simulink model "schemes"  (R2019b)
settings: Solver=VariableStepAuto  StartTime=0.0  StopTime=10.0  RelTol=1e-3
undefined symbols (not defined in the file): Ki, Kp
settings Model: Creator=joaotiagoalmeida  LastModifiedBy=joaotiagoalmeida

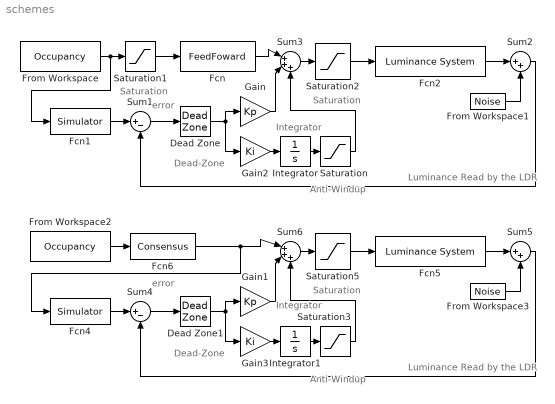
== system schemes ==
  note: Anti-Windup
  note: Dead-Zone
  note: Saturation
  note: Saturation
  note: error
  note: Luminance Read by the LDR
  note: Integrator
  note: error
  note: Luminance Read by the LDR
  note: Anti-Windup
  note: Saturation
  note: Dead-Zone
  note: Integrator
  Dead Zone : DeadZone  SaturateOnIntegerOverflow=on
  Dead Zone1 : DeadZone  SaturateOnIntegerOverflow=on
  Fcn : Fcn  Expr=FeedFoward
  Fcn1 : Fcn  Expr=Simulator
  Fcn2 : Fcn  Expr=Luminance System
  Fcn4 : Fcn  Expr=Simulator
  Fcn5 : Fcn  Expr=Luminance System
  Fcn6 : Fcn  Expr=Consensus
  From Workspace : FromWorkspace  VariableName=Occupancy  OutDataTypeStr=double  SampleTime=0  OutputAfterFinalValue=Cyclic repetition
  From Workspace1 : FromWorkspace  VariableName=Noise  OutDataTypeStr=double  SampleTime=0  OutputAfterFinalValue=Cyclic repetition
  From Workspace2 : FromWorkspace  VariableName=Occupancy  OutDataTypeStr=double  SampleTime=0  OutputAfterFinalValue=Cyclic repetition
  From Workspace3 : FromWorkspace  VariableName=Noise  OutDataTypeStr=double  SampleTime=0  OutputAfterFinalValue=Cyclic repetition
  Gain : Gain  Gain=Kp
  Gain1 : Gain  Gain=Kp
  Gain2 : Gain  Gain=Ki
  Gain3 : Gain  Gain=Ki
  Integrator : Integrator
  Integrator1 : Integrator
  Saturation{,1..3,5} (5 alike) : Saturate
  Sum1 : Sum  Inputs=|+-
  Sum2 : Sum  Inputs=|++
  Sum3 : Sum  Inputs=|+++
  Sum4 : Sum  Inputs=|+-
  Sum5 : Sum  Inputs=|++
  Sum6 : Sum  Inputs=|+++
  wires:
  Fcn1/1 -> Sum1/1
  Sum1/1 -> Dead Zone/1
  Dead Zone/1 -> Gain2/1, Gain/1
  From Workspace/1 -> Fcn1/1, Saturation1/1
  Fcn/1 -> Sum3/1
  Sum3/1 -> Saturation2/1
  Saturation/1 -> Sum3/3
  Saturation1/1 -> Fcn/1
  Gain/1 -> Sum3/2
  Saturation2/1 -> Fcn2/1
  Fcn2/1 -> Sum2/1
  From Workspace1/1 -> Sum2/2
  Sum2/1 -> Sum1/2
  Gain2/1 -> Integrator/1
  Integrator/1 -> Saturation/1
  Saturation3/1 -> Sum6/3
  Sum5/1 -> Sum4/2
  Fcn6/1 -> Fcn4/1, Sum6/1
  Fcn4/1 -> Sum4/1
  Saturation5/1 -> Fcn5/1
  Sum6/1 -> Saturation5/1
  Dead Zone1/1 -> Gain3/1, Gain1/1
  Fcn5/1 -> Sum5/1
  Sum4/1 -> Dead Zone1/1
  Gain1/1 -> Sum6/2
  From Workspace3/1 -> Sum5/2
  Gain3/1 -> Integrator1/1
  Integrator1/1 -> Saturation3/1
  From Workspace2/1 -> Fcn6/1
